simulink model "MOD5Counter"  (R2020b)
settings: Solver=VariableStepAuto  StartTime=0.0  StopTime=2  RelTol=1e-3
settings Model: EnablePacing=on  Creator=BIDITA PAUL  LastModifiedBy=BIDITA PAUL

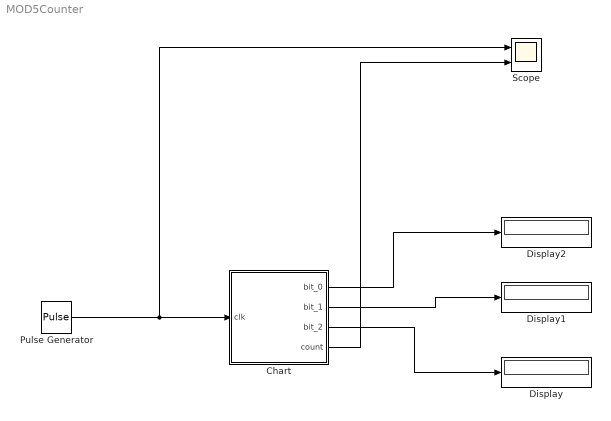
== system MOD5Counter ==
  Chart : Stateflow chart  TreatAsAtomicUnit=on
  Display : Display
  Display1 : Display
  Display2 : Display
  Pulse Generator : DiscretePulseGenerator  PulseType=Time based  Period=0.2  PulseWidth=50
  Scope : Scope  NumInputPorts=2
  wires:
  Pulse Generator/1 -> Scope/1, Chart/1(clk)
  Chart/1(bit_0) -> Display2/1
  Chart/2(bit_1) -> Display1/1
  Chart/3(bit_2) -> Display/1
  Chart/4(count) -> Scope/2

== stateflow chart MOD5Counter/Chart ==
  state STATE0
    entry:
    count =0;
    [count bit_0 bit_1 bit_2]=changeState(count, clk);
    exit:
    count = count +1;
  state STATE1
    entry:
    [count bit_0 bit_1 bit_2] = changeState(count,clk);
    exit:
    count = count+1;
  state STATE5
    entry:
    [count bit_0 bit_1 bit_2] = changeState(count, clk);
    exit:
    count = count +1;
  state STATE3
    entry:
    [count bit_0 bit_1 bit_2] = changeState(count,clk);
    exit:
    count = count +1;
  state STATE2
    entry:
    [count bit_0 bit_1 bit_2] = changeState(count,clk);
    exit:
    count = count +1;
  (default) -> STATE0
  STATE5 -> STATE0 : after(2,sec)
  STATE0 -> STATE1 : after(2, sec)
  STATE1 -> STATE2 : after(2,sec)
  STATE3 -> STATE5 : after(2,sec)
  STATE2 -> STATE3 : after(2,sec)
  data: ct function_input; ct function_output; b_0 function_output; b_1 function_output; b_2 function_output; clock function_input; clk input; bit_0 output; bit_1 output; bit_2 output; count output
  function [ct,b_0,b_1,b_2]= changeState(ct, clock):
    | function [ct,b_0,b_1,b_2]= changeState(ct, clock)
    | if clock == 1
    |     switch(ct)
    |         case ct==0
    |             b_0 = 0;
    |             b_1 = 0;
    |             b_2 = 0;
    |         case ct==1
    |             b_0 = 1;
    |             b_1 = 0;
    |             b_2 = 0;
    |         case ct==2 
    |             b_0 = 0;
    |             b_1 = 1;
    |             b_2 = 0;
    |         case ct==3
    |             b_0 = 1;
    |             b_1 = 1;
    |             b_2 = 0;
    |         case ct==4 
    |             b_0 = 0;
    |             b_1 = 0;
    |             b_2 = 1;
    |         otherwise
    |     end
    | end
    | end
